simulink model "Taller_Doblejaula_JD_Generador"  (R2023a)
settings: Solver=VariableStepAuto  StartTime=0.0  StopTime=2  MaxStep=1e-4  RelTol=1e-4
libraries: spsSeriesRLCBranchLib x3, spsAsynchronousMachineSIUnitsLib x1, spsGroundLib x1, spsMeanLib x1, spsRMSLib x1, spsThreePhaseSourceLib x1, spspowerguiLib x1
settings Model: Creator=Juan David Garcia  LastModifiedBy=Juan David
settings OptimizationCC: ReuseModelBlockBuffer=off

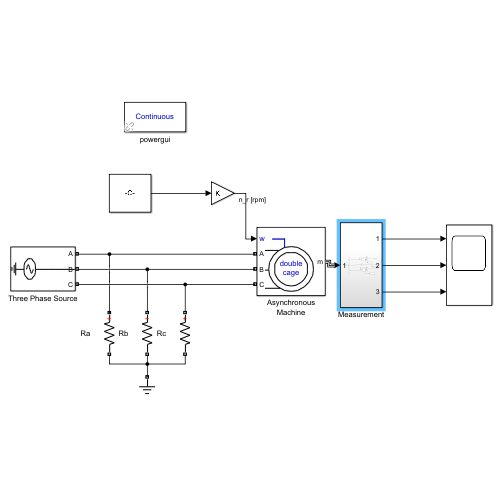
[thumbnail: Simulink's stored preview of the top-level diagram]
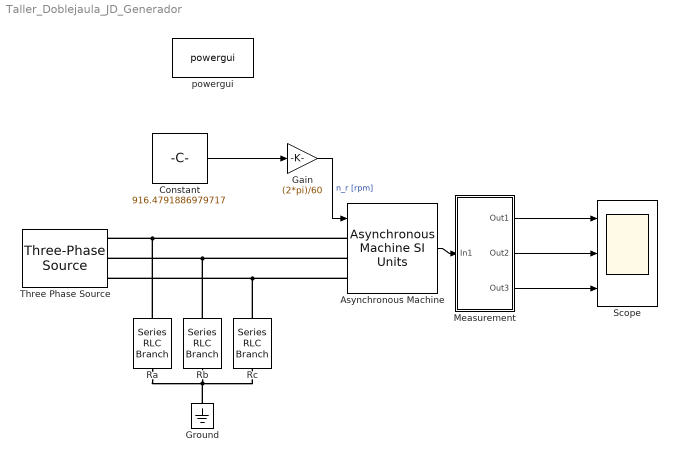
== system Taller_Doblejaula_JD_Generador ==
  Asynchronous Machine : spsAsynchronousMachineSIUnitsLib/Asynchronous Machine SI Units  RotorType=Double squirrel-cage  PresetModel=No  MechanicalLoad=Speed w  ShowDetailedParameters=on  ReferenceFrame=Synchronous  Units=SI  MeasurementBus=off  NominalParameters=[4.5e+04 660 60]  VoltageRatio=1  Stator=[0.5892 0.0009039]  Rotor=[0.832 0.0014960]  Cage1=[0.3492 0.004203]  Cage2=[0.3503 0.0009039]  Lm=0.03502  Mechanical=[(3.25+0.05) 0 4]  PolePairs=4  InitialConditions=[1 0 0 0 0 0 0 0]  SimulateSaturation=off  Saturation=[14.03593122, 27.81365428, 53.79336849, 72.68890987, 97.98006896, 148.6815601, 215.7428561, 302.9841135, 428.7778367 ; 230, 322, 414, 460, 506, 552, 598, 644, 690]  LoadFlowParameters=1492000  TsPowergui=0  TsBlock=-1  IterativeModel=Trapezoidal non iterative  IterativeDiscreteModel=Trapezoidal non iterative  Pmec=1.492e+006
  Constant : Constant  Value=916.4791886979717
  Gain : Gain  Gain=(2*pi)/60
  Ground : spsGroundLib/Ground  LConnTagsString=a
  Measurement : Subsystem
  Ra : spsSeriesRLCBranchLib/Series RLC Branch  LConnTagsString=__new0  RConnTagsString=__new0  BranchType=R  Resistance=10  Inductance=1e-3  SetiL0=off  InitialCurrent=0  Capacitance=1e-6  Setx0=off  InitialVoltage=0  Measurements=None
  Rb : spsSeriesRLCBranchLib/Series RLC Branch  LConnTagsString=__new0  RConnTagsString=__new0  BranchType=R  Resistance=10  Inductance=1e-3  SetiL0=off  InitialCurrent=0  Capacitance=1e-6  Setx0=off  InitialVoltage=0  Measurements=None
  Rc : spsSeriesRLCBranchLib/Series RLC Branch  LConnTagsString=__new0  RConnTagsString=__new0  BranchType=R  Resistance=10  Inductance=1e-3  SetiL0=off  InitialCurrent=0  Capacitance=1e-6  Setx0=off  InitialVoltage=0  Measurements=None
  Scope : Scope  NumInputPorts=3
  Three Phase Source : spsThreePhaseSourceLib/Three-Phase Source  InternalConnection=Yg  VoltagePhases=off  Voltage=660  PhaseAngle=0  Voltage_phases=[25e3 25e3 25e3]/sqrt(3)  PhaseAngles_phases=[0 -120 +120]  Frequency=60  NonIdealSource=off  SpecifyImpedance=off  Resistance=0.8929  Inductance=16.58e-3  ShortCircuitLevel=100e6  BaseVoltage=25e3  XRratio=7  BusType=swing  Pref=10e3  Qref=0  Prefabc=[10e3, 10e3, 10e3]  Qrefabc=[0, 0, 0]  Qmin=-inf  Qmax=inf
  powergui : spspowerguiLib/powergui  Priority=1  SimulationMode=Continuous  SampleTime=50e-6  frequency=60  Iterations=50  frequencyindice=60  Pbase=100e6  ErrMax=1e-4  UnitsV=kV  UnitsW=MW  buscounter=0  FunctionMessages=off  echomessages=off  EnableUseOfTLC=off  CurrentSourceSwitches=off  DisableSnubberDevices=off  DisableRonSwitches=off  DisableVfSwitches=off  DisplayEquations=off  AutomaticDiscreteSolvers=off  SolverType=Tustin/Backward Euler (TBE)  Interpol=off  ExternalGateDelay=off  methode=off  Ts=100  x0status=blocks  SPID=on  SwTol=0  HookPort=off  NonlinearTolerance=1e-4  nMaxIteration=100  ContinueOnMaxIteration=off  RestoreLinks=warning  ResistiveCurrentMeasurement=off  Frange=[0:2:500]  Ylog=off  Xlog=on  ShowGrid=off  save=off  variable=ZData  structure=0  ZoomFFT=off  StartTime=0.0  cycles=1  DisplayStyle=1  fundamental=60  FreqAxis=off  MaxFrequency=1000  frequencyindicesteady=1  RmsSteady=1  display=off
  wires:
  Measurement/2(Out2) -> Scope/2
  Measurement/1(Out1) -> Scope/1
  Measurement/3(Out3) -> Scope/3
  Asynchronous Machine/1 -> Measurement/1(In1)
  Constant/1 -> Gain/1
  Gain/1 -> Asynchronous Machine/1  "n_r [rpm]"
  connections:
  Asynchronous Machine/LConn1 -- Ra/LConn1 -- Three Phase Source/RConn1
  Asynchronous Machine/LConn2 -- Rb/LConn1 -- Three Phase Source/RConn2
  Asynchronous Machine/LConn3 -- Rc/LConn1 -- Three Phase Source/RConn3
  Ra/RConn1 -- Ground/LConn1 -- Rb/RConn1 -- Rc/RConn1

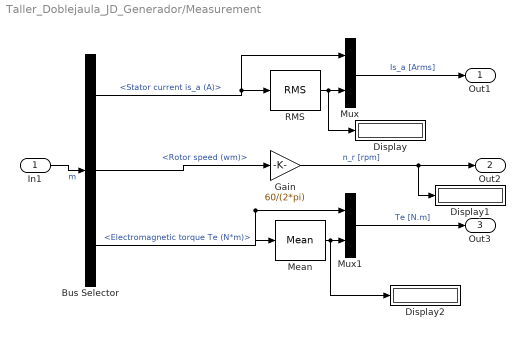
== system Taller_Doblejaula_JD_Generador/Measurement ==
  In1 : Inport
  Bus Selector : BusSelector  OutputSignals=Stator measurements.Stator current is_a (A),Mechanical.Rotor speed (wm),Mechanical.Electromagnetic torque Te (N*m)
  Display : Display
  Display1 : Display
  Display2 : Display
  Gain : Gain  Gain=60/(2*pi)
  Mean : spsMeanLib/Mean  Freq=60  Vinit=815.28  Ts=0
  Mux : Mux  Inputs=2
  Mux1 : Mux  Inputs=2
  RMS : spsRMSLib/RMS  TrueRMS=on  Freq=60  RMSInit=203.45  Ts=0
  Out1 : Outport
  Out2 : Outport  Port=2
  Out3 : Outport  Port=3
  wires:
  Bus Selector/3 -> Mean/1, Mux1/1  "<Electromagnetic torque Te (N*m)>"
  Bus Selector/2 -> Gain/1  "<Rotor speed (wm)>"
  Mux1/1 -> Out3/1  "Te [N.m]"
  Mean/1 -> Display2/1, Mux1/2
  Bus Selector/1 -> Mux/1, RMS/1  "<Stator current is_a (A)>"
  RMS/1 -> Display/1, Mux/2
  Gain/1 -> Display1/1, Out2/1  "n_r [rpm]"
  In1/1 -> Bus Selector/1  "m"
  Mux/1 -> Out1/1  "Is_a [Arms]"
